simulink model "IKs"  (Simulink 6.4)
settings: Solver=ode15s  StartTime=0.0  StopTime=sim_time  MaxStep=1e-3  MinStep=1e-7  RelTol=1e-4  AbsTol=1e-4
values from neighbouring files (symbols this model uses):
  C10o = 0    [parametersIKs.m]
  C11o = 0    [parametersIKs.m]
  C12o = 0    [parametersIKs.m]
  C13o = 0    [parametersIKs.m]
  C14o = 0    [parametersIKs.m]
  C15o = 0    [parametersIKs.m]
  C1o = 0.0015    [parametersIKs.m]
  C2o = 0.0244    [parametersIKs.m]
  C3o = 0.1494    [parametersIKs.m]
  C4o = 0.4071    [parametersIKs.m]
  C5o = 0.4161    [parametersIKs.m]
  C6o = 1-(C1o+C2o+C3o+C4o+C5o+C7o+C8o+C9o+C10o+C11o+C12o+C13o+C14o+C15o+O1o+O2o)    (= 0)    [parametersIKs.m]
  C7o = 0.0001    [parametersIKs.m]
  C8o = 0.0006    [parametersIKs.m]
  C9o = 0.0008    [parametersIKs.m]
  Caio = 1e-4    (= 0.0001)    [parametersIKs.m]
  EKs = -.0724    (= -0.0724)    [parametersIKs.m]
  F = 96485    [parametersIKs.m]
  GKsmax = 12e-9    (= 1.2e-08)    [parametersIKs.m]
  Ki = 141.2    [parametersIKs.m]
  Ko = 5.4    [parametersIKs.m]
  Nai = 10    [parametersIKs.m]
  Nao = 136    [parametersIKs.m]
  O1o = 0    [parametersIKs.m]
  O2o = 0    [parametersIKs.m]
  parexp = [8.77428657562 14.5254161368 737.410218653 97.0358106262 55.2458593549 0.320617276092 1.59085959902 0.0204263579193 0.039871941954 -0.110152581851 -0.0694163712948 -0.0481456461144 ... (20 elements, 1x20)]    [parottimiCTRL.mat]    (also in parottimiISO.mat = [13.85 14.4317602151 747.77084772 93.2952865314 46.182758087)
  pNaK = 0.01833    [parametersIKs.m]
  R = 8.314    [parametersIKs.m]
  T = 310.0    (= 310)    [parametersIKs.m]
  Vcost = 1000    [parametersIKs.m]
  x = 10e-3    (= 0.01)    [parametersIKs.m]
libraries: simulink x2
settings Model: LastModifiedBy=Stefano Severi
settings SolverCC: InitialStep=1e-5
settings DataIOCC: LimitDataPoints=off  TimeSaveName=t

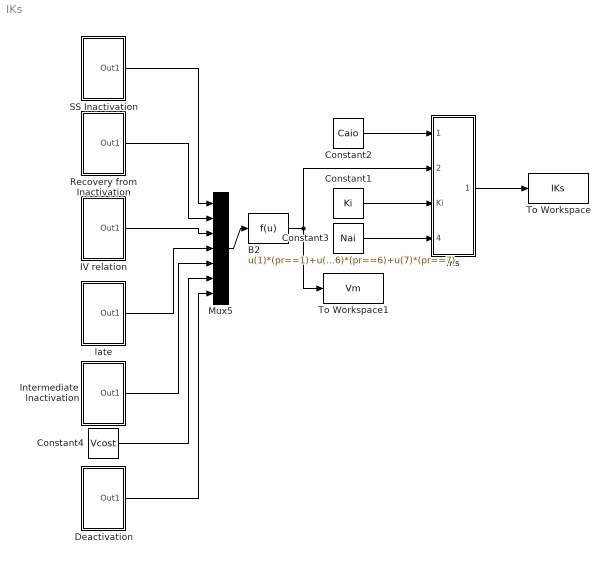
== system IKs ==
  B2 : Fcn  Expr=u(1)*(pr==1)+u(2)*(pr==2)+u(3)*(pr==3)+u(4)*(pr==4)+u(5)*(pr==5)+u(6)*(pr==6)+u(7)*(pr==7)
  Constant1 : Constant  Value=Ki  OutDataType=sfix(16)  ConRadixGroup=Use specified scaling  OutScaling=2^0  SampleTime=inf  FramePeriod=inf
  Constant2 : Constant  Value=Caio  OutDataType=sfix(16)  ConRadixGroup=Use specified scaling  OutScaling=2^0  SampleTime=inf  FramePeriod=inf
  Constant3 : Constant  Value=Nai  OutDataType=sfix(16)  ConRadixGroup=Use specified scaling  OutScaling=2^0  SampleTime=inf  FramePeriod=inf
  Constant4 : Constant  Value=Vcost  OutDataType=sfix(16)  ConRadixGroup=Use specified scaling  OutScaling=2^0  SampleTime=inf  FramePeriod=inf
  Deactivation : Subsystem
  IKs : Subsystem
  IV relation : Subsystem
  Intermediate Inactivation : Subsystem
  Mux5 : Mux  Inputs=7
  Recovery from Inactivation : Subsystem
  SS Inactivation : Subsystem
  To Workspace : ToWorkspace  VariableName=IKs  SampleTime=-1  SaveFormat=Array
  To Workspace1 : ToWorkspace  VariableName=Vm  SampleTime=-1  SaveFormat=Array
  late : Subsystem
  wires:
  IKs/1(Out1) -> To Workspace/1
  Constant2/1 -> IKs/1(Cai)
  Constant1/1 -> IKs/3(Ki)
  Constant3/1 -> IKs/4(Nai)
  Mux5/1 -> B2/1
  late/1(Out1) -> Mux5/4
  Intermediate Inactivation/1(Out1) -> Mux5/5
  SS Inactivation/1(Out1) -> Mux5/1
  Recovery from Inactivation/1(Out1) -> Mux5/2
  IV relation/1(Out1) -> Mux5/3
  B2/1 -> IKs/2(Vm), To Workspace1/1
  Constant4/1 -> Mux5/6
  Deactivation/1(Out1) -> Mux5/7

== system IKs/Deactivation ==
  Sum1 : Sum  Inputs=|+-  SaturateOnIntegerOverflow=on  InputSameDT=on
  To Workspace : ToWorkspace  VariableName=vm6  SampleTime=-1  SaveFormat=Array
  activation : Step  Time=3000e-3  Before=-0.04  After=.02  SampleTime=0
  activation1 : Step  Time=6000e-3  After=.02-x  SampleTime=0
  Out1 : Outport
  wires:
  activation/1 -> Sum1/1
  activation1/1 -> Sum1/2
  Sum1/1 -> Out1/1, To Workspace/1

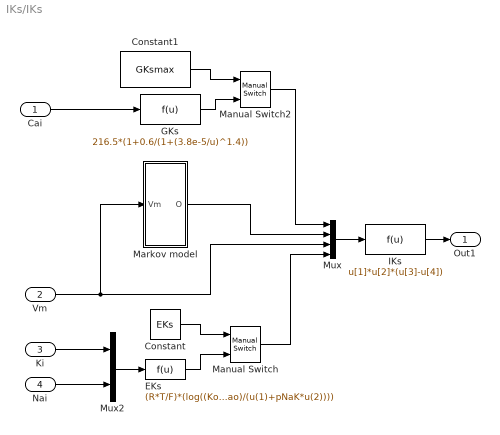
== system IKs/IKs ==
  Cai : Inport
  Vm : Inport  Port=2
  Ki : Inport  Port=3
  Nai : Inport  Port=4
  Constant : Constant  Value=EKs  OutDataType=sfix(16)  ConRadixGroup=Use specified scaling  OutScaling=2^0  SampleTime=inf  FramePeriod=inf
  Constant1 : Constant  Value=GKsmax  OutDataType=sfix(16)  ConRadixGroup=Use specified scaling  OutScaling=2^0  SampleTime=inf  FramePeriod=inf
  EKs : Fcn  Expr=(R*T/F)*(log((Ko+pNaK*Nao)/(u(1)+pNaK*u(2))))
  GKs : Fcn  Expr=216.5*(1+0.6/(1+(3.8e-5/u)^1.4))
  IKs : Fcn  Expr=u[1]*u[2]*(u[3]-u[4])
  Manual Switch : simulink/Signal Routing/Manual Switch  SystemSampleTime=-1  sw=1  action=0
  Manual Switch2 : simulink/Signal Routing/Manual Switch  SystemSampleTime=-1  sw=1  action=0
  Markov model : Subsystem
  Mux : Mux
  Mux2 : Mux  Inputs=2
  Out1 : Outport
  wires:
  Cai/1 -> GKs/1
  Markov model/1(O) -> Mux/2
  Vm/1 -> Markov model/1(Vm), Mux/3
  Mux/1 -> IKs/1
  Mux2/1 -> EKs/1
  Ki/1 -> Mux2/1
  Nai/1 -> Mux2/2
  IKs/1 -> Out1/1
  Manual Switch/1 -> Mux/4
  Constant/1 -> Manual Switch/1
  EKs/1 -> Manual Switch/2
  Constant1/1 -> Manual Switch2/1
  GKs/1 -> Manual Switch2/2
  Manual Switch2/1 -> Mux/1

== system IKs/IV relation ==
  Sum1 : Sum  Inputs=|+-  SaturateOnIntegerOverflow=on  InputSameDT=on
  To Workspace : ToWorkspace  VariableName=vm3  SampleTime=-1  SaveFormat=Array
  activation : Step  Time=3000e-3  Before=-0.04  After=x  SampleTime=0
  activation1 : Step  Time=6000e-3  After=x+30e-3  SampleTime=0
  Out1 : Outport
  wires:
  activation/1 -> Sum1/1
  activation1/1 -> Sum1/2
  Sum1/1 -> Out1/1, To Workspace/1

== system IKs/Intermediate Inactivation ==
  Step : Step  Time=50e-3  Before=-0.14  After=-0.02  SampleTime=0
  Step1 : Step  Time=50e-3+x  After=0.12  SampleTime=0
  Step2 : Step  Time=50e-3+x+20e-3  After=0.12  SampleTime=0
  Step3 : Step  Time=50e-3+x+40e-3  After=0.12  SampleTime=0
  Sum1 : Sum  Inputs=|+-+-  SaturateOnIntegerOverflow=on  InputSameDT=on
  To Workspace : ToWorkspace  VariableName=vm5  SampleTime=-1  SaveFormat=Array
  Out1 : Outport
  wires:
  Sum1/1 -> Out1/1, To Workspace/1
  Step3/1 -> Sum1/4
  Step2/1 -> Sum1/3
  Step1/1 -> Sum1/2
  Step/1 -> Sum1/1

== system IKs/Recovery from Inactivation ==
  Step : Step  Time=50e-3  Before=-0.04  After=0.02  SampleTime=0
  Step1 : Step  Time=3050e-3  After=0.1  SampleTime=0
  Step2 : Step  Time=3050e-3+x  After=0.1  SampleTime=0
  Step3 : Step  Time=3050e-3+x+3000e-3  After=0.1  SampleTime=0
  Sum1 : Sum  Inputs=|+-+-  SaturateOnIntegerOverflow=on  InputSameDT=on
  To Workspace1 : ToWorkspace  VariableName=vm2  SampleTime=-1  SaveFormat=Array
  Out1 : Outport
  wires:
  Step/1 -> Sum1/1
  Step1/1 -> Sum1/2
  Step2/1 -> Sum1/3
  Step3/1 -> Sum1/4
  Sum1/1 -> Out1/1, To Workspace1/1

== system IKs/SS Inactivation ==
  Sum2 : Sum  Inputs=|++-  SaturateOnIntegerOverflow=on  InputSameDT=on
  inactivation : Step  Time=50e-3  Before=-0.14  After=x  SampleTime=0
  inactivation1 : Step  Time=550e-3  After=-0.02-x  SampleTime=0
  inactivation2 : Step  Time=570e-3  After=+0.12  SampleTime=0
  Out1 : Outport
  wires:
  inactivation/1 -> Sum2/1
  inactivation1/1 -> Sum2/2
  inactivation2/1 -> Sum2/3
  Sum2/1 -> Out1/1

== system IKs/late ==
  Sum1 : Sum  Inputs=|+-+-  SaturateOnIntegerOverflow=on  InputSameDT=on
  To Workspace : ToWorkspace  VariableName=vm4  SampleTime=-1  SaveFormat=Array
  activation : Step  Time=50e-3  Before=-0.14  After=-0.02  SampleTime=0
  activation1 : Step  Time=1050e-3  After=0.12  SampleTime=0
  activation2 : Step  Time=2050e-3  After=0.120  SampleTime=0
  activation3 : Step  Time=3050e-3  After=0.12  SampleTime=0
  Out1 : Outport
  wires:
  activation/1 -> Sum1/1
  activation1/1 -> Sum1/2
  Sum1/1 -> Out1/1, To Workspace/1
  activation2/1 -> Sum1/3
  activation3/1 -> Sum1/4

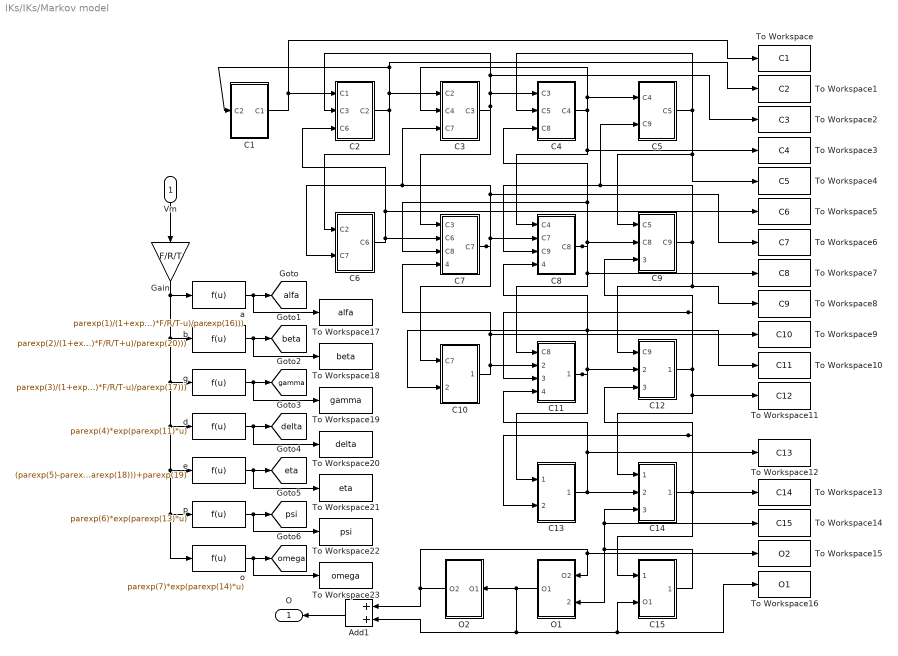
== system IKs/IKs/Markov model ==
  Vm : Inport  Orientation=down
  Add1 : Sum  Orientation=left  OutScaling=2^-10
  C1 : Subsystem
  C10 : Subsystem
  C11 : Subsystem
  C12 : Subsystem
  C13 : Subsystem
  C14 : Subsystem
  C15 : Subsystem
  C2 : Subsystem
  C3 : Subsystem
  C4 : Subsystem
  C5 : Subsystem
  C6 : Subsystem
  C7 : Subsystem
  C8 : Subsystem
  C9 : Subsystem
  Gain : Gain  Orientation=down  Gain=F/R/T
  O1 : Subsystem  Orientation=left
  O2 : Subsystem  Orientation=left
  To Workspace : ToWorkspace  VariableName=C1  SampleTime=-1  SaveFormat=Array
  To Workspace1 : ToWorkspace  VariableName=C2  SampleTime=-1  SaveFormat=Array
  To Workspace10 : ToWorkspace  VariableName=C11  SampleTime=-1  SaveFormat=Array
  To Workspace11 : ToWorkspace  VariableName=C12  SampleTime=-1  SaveFormat=Array
  To Workspace12 : ToWorkspace  VariableName=C13  SampleTime=-1  SaveFormat=Array
  To Workspace13 : ToWorkspace  VariableName=C14  SampleTime=-1  SaveFormat=Array
  To Workspace14 : ToWorkspace  VariableName=C15  SampleTime=-1  SaveFormat=Array
  To Workspace15 : ToWorkspace  VariableName=O2  SampleTime=-1  SaveFormat=Array
  To Workspace16 : ToWorkspace  VariableName=O1  SampleTime=-1  SaveFormat=Array
  To Workspace17 : ToWorkspace  VariableName=alfa  SampleTime=-1  SaveFormat=Array
  To Workspace18 : ToWorkspace  VariableName=beta  SampleTime=-1  SaveFormat=Array
  To Workspace19 : ToWorkspace  VariableName=gamma  SampleTime=-1  SaveFormat=Array
  To Workspace2 : ToWorkspace  VariableName=C3  SampleTime=-1  SaveFormat=Array
  To Workspace20 : ToWorkspace  VariableName=delta  SampleTime=-1  SaveFormat=Array
  To Workspace21 : ToWorkspace  VariableName=eta  SampleTime=-1  SaveFormat=Array
  To Workspace22 : ToWorkspace  VariableName=psi  SampleTime=-1  SaveFormat=Array
  To Workspace23 : ToWorkspace  VariableName=omega  SampleTime=-1  SaveFormat=Array
  To Workspace3 : ToWorkspace  VariableName=C4  SampleTime=-1  SaveFormat=Array
  To Workspace4 : ToWorkspace  VariableName=C5  SampleTime=-1  SaveFormat=Array
  To Workspace5 : ToWorkspace  VariableName=C6  SampleTime=-1  SaveFormat=Array
  To Workspace6 : ToWorkspace  VariableName=C7  SampleTime=-1  SaveFormat=Array
  To Workspace7 : ToWorkspace  VariableName=C8  SampleTime=-1  SaveFormat=Array
  To Workspace8 : ToWorkspace  VariableName=C9  SampleTime=-1  SaveFormat=Array
  To Workspace9 : ToWorkspace  VariableName=C10  SampleTime=-1  SaveFormat=Array
  a : Fcn  Expr=parexp(1)/(1+exp((parexp(8)*F/R/T-u)/parexp(16)))
  b : Fcn  Expr=parexp(2)/(1+exp((-parexp(9)*F/R/T+u)/parexp(20)))
  d : Fcn  Expr=parexp(4)*exp(parexp(11)*u)
  e : Fcn  Expr=(parexp(5)-parexp(19))/(1+exp((-parexp(12)*F/R/T+u)/parexp(18)))+parexp(19)
  g : Fcn  Expr=parexp(3)/(1+exp((parexp(10)*F/R/T-u)/parexp(17)))
  o : Fcn  Expr=parexp(7)*exp(parexp(14)*u)
  p : Fcn  Expr=parexp(6)*exp(parexp(13)*u)
  O : Outport  Orientation=left
  tag scope: alfa=global, beta=global, delta=global, eta=global, gamma=global, omega=global, psi=global
  wires:
  C1/1(C1) -> C2/1(C1), To Workspace/1
  C2/1(C2) -> C3/1(C2), C1/1(C2), To Workspace1/1, C6/1(C2)
  C3/1(C3) -> C4/1(C3), C2/2(C3), To Workspace2/1, C7/1(C3)
  C4/1(C4) -> C3/2(C4), C5/1(C4), C8/1(C4), To Workspace3/1
  C5/1(C5) -> C4/2(C5), C9/1(C5), To Workspace4/1
  C6/1(C6) -> C7/2(C6), C2/3(C6), To Workspace5/1
  C7/1(C7) -> C8/2(C7), C3/3(C7), C6/2(C7), To Workspace6/1, C10/1(C7)
  C8/1(C8) -> C4/3(C8), C7/3(C8), C9/2(C8), C11/1(C8), To Workspace7/1
  C9/1(C9) -> C5/2(C9), C8/3(C9), C12/1(C9), To Workspace8/1
  C10/1(C10) -> C11/2(C10), C7/4(C10), To Workspace9/1
  C11/1(C11) -> C8/4(C11), C10/2(C11), To Workspace10/1, C12/2(C11), C13/1(C11)
  C12/1(C12) -> C9/3(C12), C11/3(C12), C14/1(C12), To Workspace11/1
  C13/1(C13) -> C14/2(C13), C11/4(C13), To Workspace12/1
  C14/1(C14) -> C12/3(C14), C13/2(C14), C15/1(C14), To Workspace13/1
  C15/1(C15) -> O1/2(C15), C14/3(C15), To Workspace14/1
  O2/1(O2) -> O1/1(O2), To Workspace15/1, Add1/1
  O1/1(O1) -> C15/2(O1), To Workspace16/1, Add1/2, O2/1(O1)
  Add1/1 -> O/1
  Gain/1 -> a/1, b/1, g/1, d/1, e/1, p/1, o/1
  a/1 -> [alfa], To Workspace17/1
  b/1 -> [beta], To Workspace18/1
  g/1 -> [gamma], To Workspace19/1
  d/1 -> [delta], To Workspace20/1
  e/1 -> [eta], To Workspace21/1
  p/1 -> [psi], To Workspace22/1
  o/1 -> [omega], To Workspace23/1
  Vm/1 -> Gain/1

== system IKs/IKs/Markov model/C1 ==
  C2 : Inport
  GKs : Fcn  Expr=4*u[1]*u[2]
  GKs1 : Fcn  Expr=u[1]*u[2]
  Integrator : Integrator  InitialCondition=C1o
  Mux : Mux  Inputs=2
  Mux1 : Mux  Inputs=2
  Sum3 : Sum  Inputs=-+  SaturateOnIntegerOverflow=on  InputSameDT=on
  C1 : Outport
  wires:
  Sum3/1 -> Integrator/1
  Integrator/1 -> C1/1, Mux/1
  GKs1/1 -> Sum3/2
  GKs/1 -> Sum3/1
  Mux/1 -> GKs/1
  [alfa] -> Mux/2
  [beta] -> Mux1/2
  Mux1/1 -> GKs1/1
  C2/1 -> Mux1/1

== system IKs/IKs/Markov model/C10 ==
  C7 : Inport
  C11 : Inport  Port=2
  GKs : Fcn  Expr=u[1]*(2*u[2]+2*u[3])
  GKs1 : Fcn  Expr=u[1]*u[2]
  GKs3 : Fcn  Expr=u[1]*u[2]
  Integrator : Integrator  InitialCondition=C10o
  Mux : Mux  Inputs=3
  Mux1 : Mux  Inputs=2
  Mux3 : Mux  Inputs=2
  Sum3 : Sum  Inputs=-++  SaturateOnIntegerOverflow=on  InputSameDT=on
  C10 : Outport
  wires:
  GKs3/1 -> Sum3/3
  GKs/1 -> Sum3/1
  C11/1 -> Mux3/1
  Mux3/1 -> GKs3/1
  [beta] -> Mux3/2
  [delta] -> Mux/3
  C7/1 -> Mux1/1
  Mux1/1 -> GKs1/1
  [gamma] -> Mux1/2
  Mux/1 -> GKs/1
  GKs1/1 -> Sum3/2
  Integrator/1 -> Mux/1, C10/1
  Sum3/1 -> Integrator/1
  [alfa] -> Mux/2

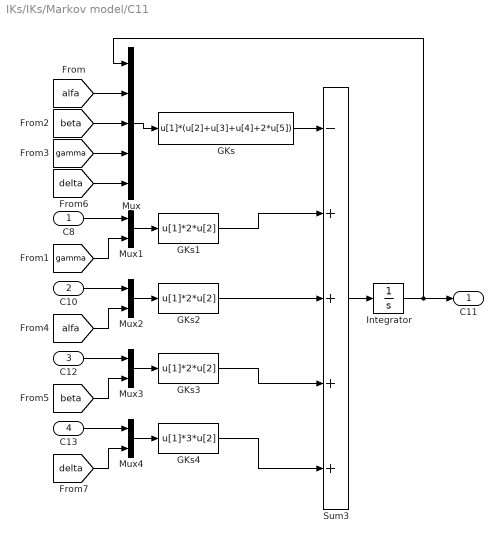
== system IKs/IKs/Markov model/C11 ==
  C8 : Inport
  C10 : Inport  Port=2
  C12 : Inport  Port=3
  C13 : Inport  Port=4
  GKs : Fcn  Expr=u[1]*(u[2]+u[3]+u[4]+2*u[5])
  GKs1 : Fcn  Expr=u[1]*2*u[2]
  GKs2 : Fcn  Expr=u[1]*2*u[2]
  GKs3 : Fcn  Expr=u[1]*2*u[2]
  GKs4 : Fcn  Expr=u[1]*3*u[2]
  Integrator : Integrator  InitialCondition=C11o
  Mux : Mux  Inputs=5
  Mux{1..4} (4 alike) : Mux  Inputs=2
  Sum3 : Sum  Inputs=-++++  SaturateOnIntegerOverflow=on  InputSameDT=on
  C11 : Outport
  wires:
  [delta] -> Mux4/2
  Mux4/1 -> GKs4/1
  C13/1 -> Mux4/1
  GKs4/1 -> Sum3/5
  [delta] -> Mux/5
  Sum3/1 -> Integrator/1
  Integrator/1 -> C11/1, Mux/1
  GKs1/1 -> Sum3/2
  Mux/1 -> GKs/1
  [alfa] -> Mux/2
  [gamma] -> Mux1/2
  Mux1/1 -> GKs1/1
  C8/1 -> Mux1/1
  [gamma] -> Mux/4
  [beta] -> Mux/3
  GKs2/1 -> Sum3/3
  [alfa] -> Mux2/2
  Mux2/1 -> GKs2/1
  C10/1 -> Mux2/1
  [beta] -> Mux3/2
  Mux3/1 -> GKs3/1
  C12/1 -> Mux3/1
  GKs/1 -> Sum3/1
  GKs3/1 -> Sum3/4

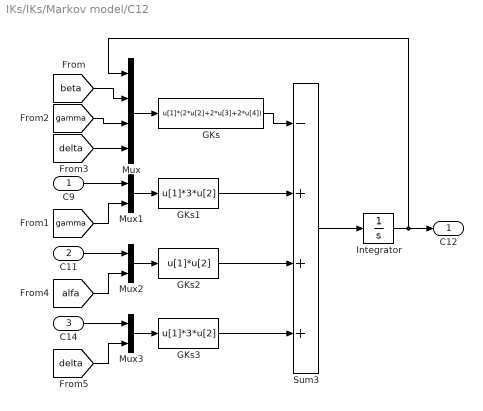
== system IKs/IKs/Markov model/C12 ==
  C9 : Inport
  C11 : Inport  Port=2
  C14 : Inport  Port=3
  GKs : Fcn  Expr=u[1]*(2*u[2]+2*u[3]+2*u[4])
  GKs1 : Fcn  Expr=u[1]*3*u[2]
  GKs2 : Fcn  Expr=u[1]*u[2]
  GKs3 : Fcn  Expr=u[1]*3*u[2]
  Integrator : Integrator  InitialCondition=C12o
  Mux : Mux
  Mux1 : Mux  Inputs=2
  Mux2 : Mux  Inputs=2
  Mux3 : Mux  Inputs=2
  Sum3 : Sum  Inputs=-+++  SaturateOnIntegerOverflow=on  InputSameDT=on
  C12 : Outport
  wires:
  GKs3/1 -> Sum3/4
  GKs/1 -> Sum3/1
  C14/1 -> Mux3/1
  Mux3/1 -> GKs3/1
  [delta] -> Mux3/2
  C11/1 -> Mux2/1
  Mux2/1 -> GKs2/1
  [alfa] -> Mux2/2
  GKs2/1 -> Sum3/3
  [gamma] -> Mux/3
  [delta] -> Mux/4
  C9/1 -> Mux1/1
  Mux1/1 -> GKs1/1
  [gamma] -> Mux1/2
  [beta] -> Mux/2
  Mux/1 -> GKs/1
  GKs1/1 -> Sum3/2
  Integrator/1 -> Mux/1, C12/1
  Sum3/1 -> Integrator/1

== system IKs/IKs/Markov model/C13 ==
  C11 : Inport
  C14 : Inport  Port=2
  GKs : Fcn  Expr=u[1]*(u[2]+3*u[3])
  GKs1 : Fcn  Expr=u[1]*u[2]
  GKs3 : Fcn  Expr=u[1]*u[2]
  Integrator : Integrator  InitialCondition=C13o
  Mux : Mux  Inputs=3
  Mux1 : Mux  Inputs=2
  Mux3 : Mux  Inputs=2
  Sum3 : Sum  Inputs=-++  SaturateOnIntegerOverflow=on  InputSameDT=on
  C13 : Outport
  wires:
  [alfa] -> Mux/2
  Sum3/1 -> Integrator/1
  Integrator/1 -> C13/1, Mux/1
  GKs1/1 -> Sum3/2
  Mux/1 -> GKs/1
  [gamma] -> Mux1/2
  Mux1/1 -> GKs1/1
  C11/1 -> Mux1/1
  [delta] -> Mux/3
  [beta] -> Mux3/2
  Mux3/1 -> GKs3/1
  C14/1 -> Mux3/1
  GKs/1 -> Sum3/1
  GKs3/1 -> Sum3/3

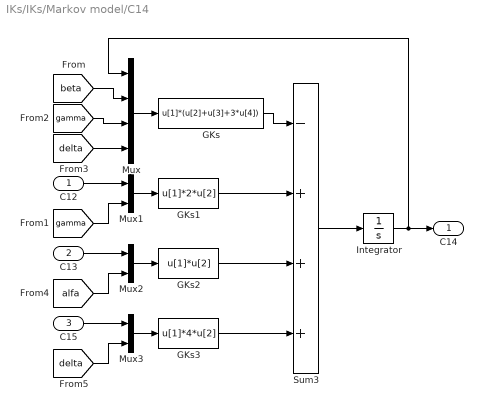
== system IKs/IKs/Markov model/C14 ==
  C12 : Inport
  C13 : Inport  Port=2
  C15 : Inport  Port=3
  GKs : Fcn  Expr=u[1]*(u[2]+u[3]+3*u[4])
  GKs1 : Fcn  Expr=u[1]*2*u[2]
  GKs2 : Fcn  Expr=u[1]*u[2]
  GKs3 : Fcn  Expr=u[1]*4*u[2]
  Integrator : Integrator  InitialCondition=C14o
  Mux : Mux
  Mux1 : Mux  Inputs=2
  Mux2 : Mux  Inputs=2
  Mux3 : Mux  Inputs=2
  Sum3 : Sum  Inputs=-+++  SaturateOnIntegerOverflow=on  InputSameDT=on
  C14 : Outport
  wires:
  Sum3/1 -> Integrator/1
  Integrator/1 -> C14/1, Mux/1
  GKs1/1 -> Sum3/2
  Mux/1 -> GKs/1
  [beta] -> Mux/2
  [gamma] -> Mux1/2
  Mux1/1 -> GKs1/1
  C12/1 -> Mux1/1
  [delta] -> Mux/4
  [gamma] -> Mux/3
  GKs2/1 -> Sum3/3
  [alfa] -> Mux2/2
  Mux2/1 -> GKs2/1
  C13/1 -> Mux2/1
  [delta] -> Mux3/2
  Mux3/1 -> GKs3/1
  C15/1 -> Mux3/1
  GKs/1 -> Sum3/1
  GKs3/1 -> Sum3/4

== system IKs/IKs/Markov model/C15 ==
  C14 : Inport
  O1 : Inport  Port=2
  GKs : Fcn  Expr=u[1]*(4*u[2]+parexp(15))
  GKs1 : Fcn  Expr=u[1]*u[2]
  GKs3 : Fcn  Expr=u[1]*u[2]
  Integrator : Integrator  InitialCondition=C15o
  Mux : Mux  Inputs=2
  Mux1 : Mux  Inputs=2
  Mux3 : Mux  Inputs=2
  Sum3 : Sum  Inputs=-++  SaturateOnIntegerOverflow=on  InputSameDT=on
  C15 : Outport
  wires:
  GKs3/1 -> Sum3/3
  GKs/1 -> Sum3/1
  O1/1 -> Mux3/1
  Mux3/1 -> GKs3/1
  [eta] -> Mux3/2
  [delta] -> Mux/2
  C14/1 -> Mux1/1
  Mux1/1 -> GKs1/1
  [gamma] -> Mux1/2
  Mux/1 -> GKs/1
  GKs1/1 -> Sum3/2
  Integrator/1 -> Mux/1, C15/1
  Sum3/1 -> Integrator/1

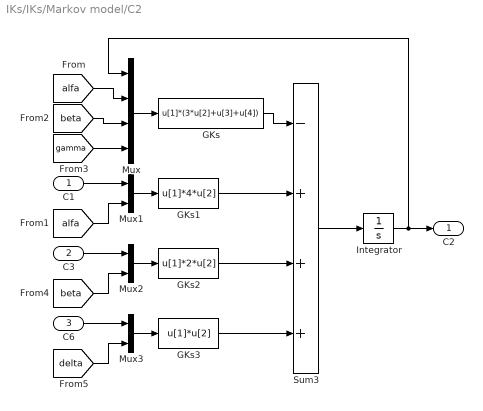
== system IKs/IKs/Markov model/C2 ==
  C1 : Inport
  C3 : Inport  Port=2
  C6 : Inport  Port=3
  GKs : Fcn  Expr=u[1]*(3*u[2]+u[3]+u[4])
  GKs1 : Fcn  Expr=u[1]*4*u[2]
  GKs2 : Fcn  Expr=u[1]*2*u[2]
  GKs3 : Fcn  Expr=u[1]*u[2]
  Integrator : Integrator  InitialCondition=C2o
  Mux : Mux
  Mux1 : Mux  Inputs=2
  Mux2 : Mux  Inputs=2
  Mux3 : Mux  Inputs=2
  Sum3 : Sum  Inputs=-+++  SaturateOnIntegerOverflow=on  InputSameDT=on
  C2 : Outport
  wires:
  Sum3/1 -> Integrator/1
  Integrator/1 -> C2/1, Mux/1
  GKs1/1 -> Sum3/2
  Mux/1 -> GKs/1
  [alfa] -> Mux/2
  [alfa] -> Mux1/2
  Mux1/1 -> GKs1/1
  C1/1 -> Mux1/1
  [gamma] -> Mux/4
  [beta] -> Mux/3
  GKs2/1 -> Sum3/3
  [beta] -> Mux2/2
  Mux2/1 -> GKs2/1
  C3/1 -> Mux2/1
  [delta] -> Mux3/2
  Mux3/1 -> GKs3/1
  C6/1 -> Mux3/1
  GKs/1 -> Sum3/1
  GKs3/1 -> Sum3/4

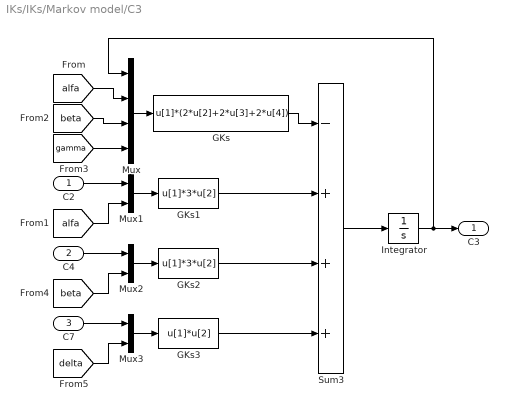
== system IKs/IKs/Markov model/C3 ==
  C2 : Inport
  C4 : Inport  Port=2
  C7 : Inport  Port=3
  GKs : Fcn  Expr=u[1]*(2*u[2]+2*u[3]+2*u[4])
  GKs1 : Fcn  Expr=u[1]*3*u[2]
  GKs2 : Fcn  Expr=u[1]*3*u[2]
  GKs3 : Fcn  Expr=u[1]*u[2]
  Integrator : Integrator  InitialCondition=C3o
  Mux : Mux
  Mux1 : Mux  Inputs=2
  Mux2 : Mux  Inputs=2
  Mux3 : Mux  Inputs=2
  Sum3 : Sum  Inputs=-+++  SaturateOnIntegerOverflow=on  InputSameDT=on
  C3 : Outport
  wires:
  GKs3/1 -> Sum3/4
  GKs/1 -> Sum3/1
  C7/1 -> Mux3/1
  Mux3/1 -> GKs3/1
  [delta] -> Mux3/2
  C4/1 -> Mux2/1
  Mux2/1 -> GKs2/1
  [beta] -> Mux2/2
  GKs2/1 -> Sum3/3
  [beta] -> Mux/3
  [gamma] -> Mux/4
  C2/1 -> Mux1/1
  Mux1/1 -> GKs1/1
  [alfa] -> Mux1/2
  [alfa] -> Mux/2
  Mux/1 -> GKs/1
  GKs1/1 -> Sum3/2
  Integrator/1 -> Mux/1, C3/1
  Sum3/1 -> Integrator/1

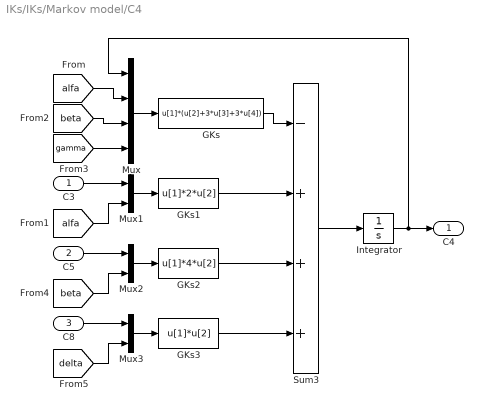
== system IKs/IKs/Markov model/C4 ==
  C3 : Inport
  C5 : Inport  Port=2
  C8 : Inport  Port=3
  GKs : Fcn  Expr=u[1]*(u[2]+3*u[3]+3*u[4])
  GKs1 : Fcn  Expr=u[1]*2*u[2]
  GKs2 : Fcn  Expr=u[1]*4*u[2]
  GKs3 : Fcn  Expr=u[1]*u[2]
  Integrator : Integrator  InitialCondition=C4o
  Mux : Mux
  Mux1 : Mux  Inputs=2
  Mux2 : Mux  Inputs=2
  Mux3 : Mux  Inputs=2
  Sum3 : Sum  Inputs=-+++  SaturateOnIntegerOverflow=on  InputSameDT=on
  C4 : Outport
  wires:
  GKs3/1 -> Sum3/4
  GKs/1 -> Sum3/1
  C8/1 -> Mux3/1
  Mux3/1 -> GKs3/1
  [delta] -> Mux3/2
  C5/1 -> Mux2/1
  Mux2/1 -> GKs2/1
  [beta] -> Mux2/2
  GKs2/1 -> Sum3/3
  [beta] -> Mux/3
  [gamma] -> Mux/4
  C3/1 -> Mux1/1
  Mux1/1 -> GKs1/1
  [alfa] -> Mux1/2
  [alfa] -> Mux/2
  Mux/1 -> GKs/1
  GKs1/1 -> Sum3/2
  Integrator/1 -> Mux/1, C4/1
  Sum3/1 -> Integrator/1

== system IKs/IKs/Markov model/C5 ==
  C4 : Inport
  C9 : Inport  Port=2
  GKs : Fcn  Expr=u[1]*(4*u[2]+4*u[3])
  GKs1 : Fcn  Expr=u[1]*u[2]
  GKs3 : Fcn  Expr=u[1]*u[2]
  Integrator : Integrator  InitialCondition=C5o
  Mux : Mux  Inputs=3
  Mux1 : Mux  Inputs=2
  Mux3 : Mux  Inputs=2
  Sum3 : Sum  Inputs=-++  SaturateOnIntegerOverflow=on  InputSameDT=on
  C5 : Outport
  wires:
  GKs3/1 -> Sum3/3
  GKs/1 -> Sum3/1
  C9/1 -> Mux3/1
  Mux3/1 -> GKs3/1
  [delta] -> Mux3/2
  [gamma] -> Mux/3
  C4/1 -> Mux1/1
  Mux1/1 -> GKs1/1
  [alfa] -> Mux1/2
  Mux/1 -> GKs/1
  GKs1/1 -> Sum3/2
  Integrator/1 -> Mux/1, C5/1
  Sum3/1 -> Integrator/1
  [beta] -> Mux/2

== system IKs/IKs/Markov model/C6 ==
  C2 : Inport
  C7 : Inport  Port=2
  GKs : Fcn  Expr=u[1]*(3*u[2]+u[3])
  GKs1 : Fcn  Expr=u[1]*u[2]
  GKs3 : Fcn  Expr=u[1]*u[2]
  Integrator : Integrator  InitialCondition=C6o
  Mux : Mux  Inputs=3
  Mux1 : Mux  Inputs=2
  Mux3 : Mux  Inputs=2
  Sum3 : Sum  Inputs=-++  SaturateOnIntegerOverflow=on  InputSameDT=on
  C6 : Outport
  wires:
  [alfa] -> Mux/2
  Sum3/1 -> Integrator/1
  Integrator/1 -> C6/1, Mux/1
  GKs1/1 -> Sum3/2
  Mux/1 -> GKs/1
  [gamma] -> Mux1/2
  Mux1/1 -> GKs1/1
  C2/1 -> Mux1/1
  [delta] -> Mux/3
  [beta] -> Mux3/2
  Mux3/1 -> GKs3/1
  C7/1 -> Mux3/1
  GKs/1 -> Sum3/1
  GKs3/1 -> Sum3/3

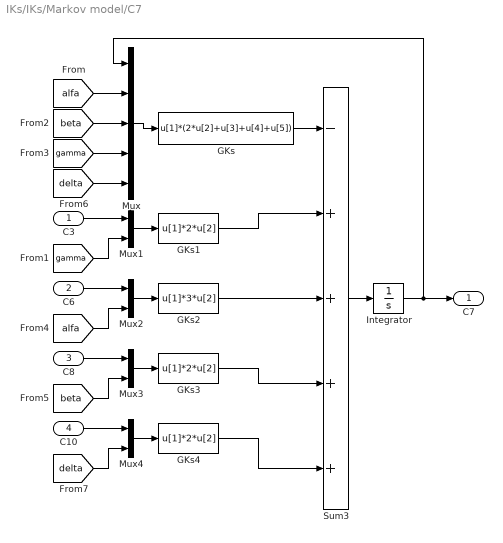
== system IKs/IKs/Markov model/C7 ==
  C3 : Inport
  C6 : Inport  Port=2
  C8 : Inport  Port=3
  C10 : Inport  Port=4
  GKs : Fcn  Expr=u[1]*(2*u[2]+u[3]+u[4]+u[5])
  GKs1 : Fcn  Expr=u[1]*2*u[2]
  GKs2 : Fcn  Expr=u[1]*3*u[2]
  GKs3 : Fcn  Expr=u[1]*2*u[2]
  GKs4 : Fcn  Expr=u[1]*2*u[2]
  Integrator : Integrator  InitialCondition=C7o
  Mux : Mux  Inputs=5
  Mux{1..4} (4 alike) : Mux  Inputs=2
  Sum3 : Sum  Inputs=-++++  SaturateOnIntegerOverflow=on  InputSameDT=on
  C7 : Outport
  wires:
  GKs3/1 -> Sum3/4
  GKs/1 -> Sum3/1
  C8/1 -> Mux3/1
  Mux3/1 -> GKs3/1
  [beta] -> Mux3/2
  C6/1 -> Mux2/1
  Mux2/1 -> GKs2/1
  [alfa] -> Mux2/2
  GKs2/1 -> Sum3/3
  [beta] -> Mux/3
  [gamma] -> Mux/4
  C3/1 -> Mux1/1
  Mux1/1 -> GKs1/1
  [gamma] -> Mux1/2
  [alfa] -> Mux/2
  Mux/1 -> GKs/1
  GKs1/1 -> Sum3/2
  Integrator/1 -> Mux/1, C7/1
  Sum3/1 -> Integrator/1
  [delta] -> Mux/5
  GKs4/1 -> Sum3/5
  C10/1 -> Mux4/1
  Mux4/1 -> GKs4/1
  [delta] -> Mux4/2

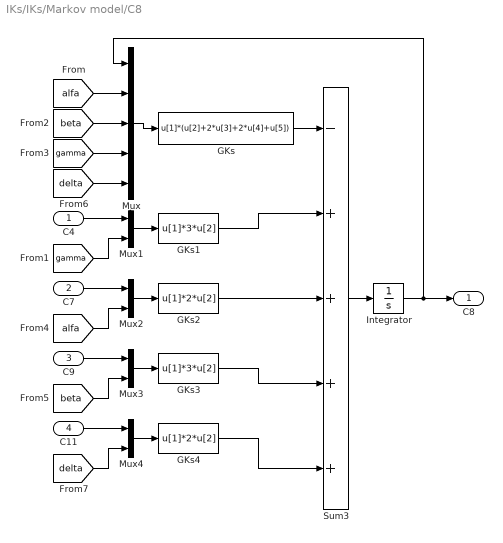
== system IKs/IKs/Markov model/C8 ==
  C4 : Inport
  C7 : Inport  Port=2
  C9 : Inport  Port=3
  C11 : Inport  Port=4
  GKs : Fcn  Expr=u[1]*(u[2]+2*u[3]+2*u[4]+u[5])
  GKs1 : Fcn  Expr=u[1]*3*u[2]
  GKs2 : Fcn  Expr=u[1]*2*u[2]
  GKs3 : Fcn  Expr=u[1]*3*u[2]
  GKs4 : Fcn  Expr=u[1]*2*u[2]
  Integrator : Integrator  InitialCondition=C8o
  Mux : Mux  Inputs=5
  Mux{1..4} (4 alike) : Mux  Inputs=2
  Sum3 : Sum  Inputs=-++++  SaturateOnIntegerOverflow=on  InputSameDT=on
  C8 : Outport
  wires:
  [delta] -> Mux4/2
  Mux4/1 -> GKs4/1
  C11/1 -> Mux4/1
  GKs4/1 -> Sum3/5
  [delta] -> Mux/5
  Sum3/1 -> Integrator/1
  Integrator/1 -> C8/1, Mux/1
  GKs1/1 -> Sum3/2
  Mux/1 -> GKs/1
  [alfa] -> Mux/2
  [gamma] -> Mux1/2
  Mux1/1 -> GKs1/1
  C4/1 -> Mux1/1
  [gamma] -> Mux/4
  [beta] -> Mux/3
  GKs2/1 -> Sum3/3
  [alfa] -> Mux2/2
  Mux2/1 -> GKs2/1
  C7/1 -> Mux2/1
  [beta] -> Mux3/2
  Mux3/1 -> GKs3/1
  C9/1 -> Mux3/1
  GKs/1 -> Sum3/1
  GKs3/1 -> Sum3/4

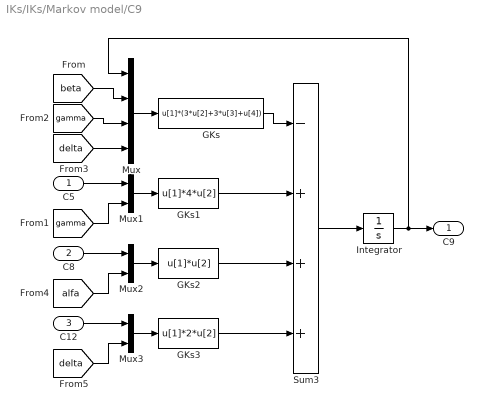
== system IKs/IKs/Markov model/C9 ==
  C5 : Inport
  C8 : Inport  Port=2
  C12 : Inport  Port=3
  GKs : Fcn  Expr=u[1]*(3*u[2]+3*u[3]+u[4])
  GKs1 : Fcn  Expr=u[1]*4*u[2]
  GKs2 : Fcn  Expr=u[1]*u[2]
  GKs3 : Fcn  Expr=u[1]*2*u[2]
  Integrator : Integrator  InitialCondition=C9o
  Mux : Mux
  Mux1 : Mux  Inputs=2
  Mux2 : Mux  Inputs=2
  Mux3 : Mux  Inputs=2
  Sum3 : Sum  Inputs=-+++  SaturateOnIntegerOverflow=on  InputSameDT=on
  C9 : Outport
  wires:
  Sum3/1 -> Integrator/1
  Integrator/1 -> C9/1, Mux/1
  GKs1/1 -> Sum3/2
  Mux/1 -> GKs/1
  [beta] -> Mux/2
  [gamma] -> Mux1/2
  Mux1/1 -> GKs1/1
  C5/1 -> Mux1/1
  [delta] -> Mux/4
  [gamma] -> Mux/3
  GKs2/1 -> Sum3/3
  [alfa] -> Mux2/2
  Mux2/1 -> GKs2/1
  C8/1 -> Mux2/1
  [delta] -> Mux3/2
  Mux3/1 -> GKs3/1
  C12/1 -> Mux3/1
  GKs/1 -> Sum3/1
  GKs3/1 -> Sum3/4

== system IKs/IKs/Markov model/O1 ==
  O2 : Inport
  C15 : Inport  Port=2
  GKs : Fcn  Expr=u[1]*(u[2]+u[3])
  GKs3 : Fcn  Expr=u[1]*u[2]
  Gain : Gain  Gain=parexp(15)
  Integrator : Integrator  InitialCondition=O1o
  Mux : Mux  Inputs=3
  Mux3 : Mux  Inputs=2
  Sum3 : Sum  Inputs=-++  SaturateOnIntegerOverflow=on  InputSameDT=on
  O1 : Outport
  wires:
  [eta] -> Mux/2
  Sum3/1 -> Integrator/1
  Integrator/1 -> O1/1, Mux/1
  Mux/1 -> GKs/1
  [psi] -> Mux/3
  [omega] -> Mux3/2
  Mux3/1 -> GKs3/1
  O2/1 -> Mux3/1
  GKs/1 -> Sum3/1
  GKs3/1 -> Sum3/3
  C15/1 -> Gain/1
  Gain/1 -> Sum3/2

== system IKs/IKs/Markov model/O2 ==
  O1 : Inport
  GKs : Fcn  Expr=u[1]*u[2]
  GKs3 : Fcn  Expr=u[1]*u[2]
  Integrator : Integrator  InitialCondition=O2o
  Mux : Mux  Inputs=2
  Mux3 : Mux  Inputs=2
  Sum3 : Sum  Inputs=-+  SaturateOnIntegerOverflow=on  InputSameDT=on
  O2 : Outport
  wires:
  GKs3/1 -> Sum3/2
  GKs/1 -> Sum3/1
  O1/1 -> Mux3/1
  Mux3/1 -> GKs3/1
  [psi] -> Mux3/2
  Mux/1 -> GKs/1
  Integrator/1 -> Mux/1, O2/1
  Sum3/1 -> Integrator/1
  [omega] -> Mux/2
